simulink subsystem "Global_2_Local_Yaw"  (R2022b)
settings: Solver=VariableStepAuto  StartTime=0.0  StopTime=10.0  RelTol=1e-3
settings Model: Creator=User  LastModifiedBy=User

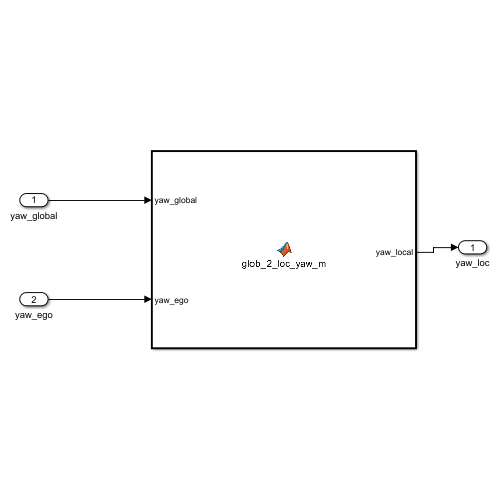
[thumbnail: Simulink's stored preview of the top-level diagram]
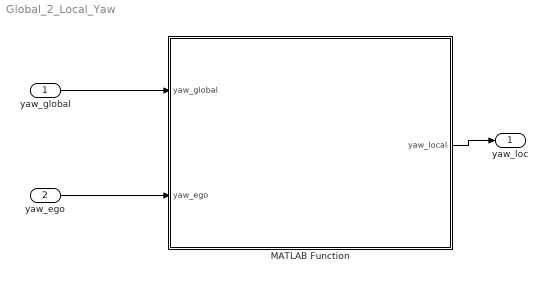
== system Global_2_Local_Yaw ==
  yaw_global : Inport
  yaw_ego : Inport  Port=2
  MATLAB Function : MATLAB Function  TreatAsAtomicUnit=on
  yaw_loc : Outport
  wires:
  yaw_global/1 -> MATLAB Function/1(yaw_global)
  yaw_ego/1 -> MATLAB Function/2(yaw_ego)
  MATLAB Function/1(yaw_local) -> yaw_loc/1

== matlab function Global_2_Local_Yaw/MATLAB Function ==
  data: yaw_global input; yaw_local output; yaw_ego input
function yaw_local = glob_2_loc_yaw_m(yaw_global, yaw_ego)
    yaw_local = glob_2_loc_yaw(yaw_global, yaw_ego);
    
end
